simulink model "controlsystems.slx"  (R2025b)
settings: Solver=VariableStepAuto  StartTime=0.0  StopTime=50  RelTol=1e-3
libraries: simulink x1
settings Model: Creator=MANAL CHATT  LastModifiedBy=MANAL CHATT

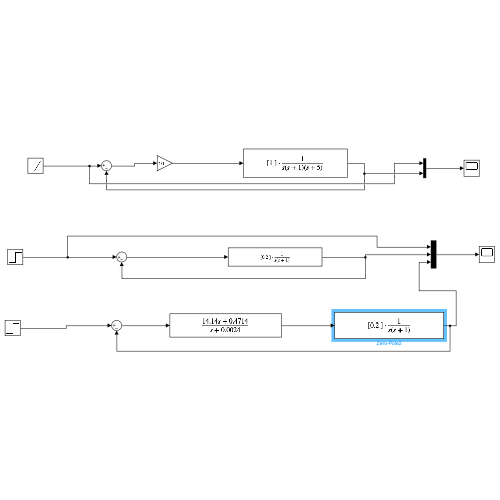
[thumbnail: Simulink's stored preview of the top-level diagram]
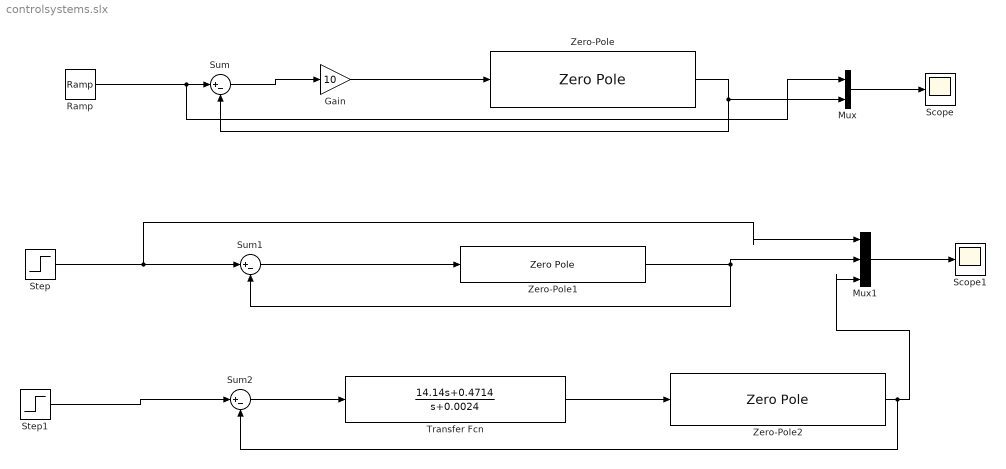
== system controlsystems.slx ==
  Gain : Gain  Gain=10
  Mux : Mux  Inputs=2
  Mux1 : Mux  Inputs=3
  Ramp : simulink/Sources/Ramp  slope=1  start=0  InitialOutput=0
  Scope : Scope
      settings: ActiveDisplayYMinimum=-6.2499999999999982  ActiveDisplayYMaximum=56.25
  Scope1 : Scope
      settings: ActiveDisplayYMinimum=-0.17289112553969113  ActiveDisplayYMaximum=1.5560201298572205
  Step : Step  SampleTime=0
  Step1 : Step  SampleTime=0
  Sum : Sum  Inputs=|+-
  Sum1 : Sum  Inputs=|+-
  Sum2 : Sum  Inputs=|+-
  Transfer Fcn : TransferFcn  Numerator=[14.14 0.4714]  Denominator=[1 0.0024]
  Zero-Pole : ZeroPole  Zeros=[]  Poles=[0 -1 -5]
  Zero-Pole1 : ZeroPole  Zeros=[]  Poles=[0 -1]  Gain=[0.2]
  Zero-Pole2 : ZeroPole  Zeros=[]  Poles=[0 -1]  Gain=[0.2]
  wires:
  Gain/1 -> Zero-Pole/1
  Zero-Pole/1 -> Mux/2, Sum/2
  Sum/1 -> Gain/1
  Mux/1 -> Scope/1
  Ramp/1 -> Mux/1, Sum/1
  Step/1 -> Mux1/1, Sum1/1
  Zero-Pole1/1 -> Sum1/2, Mux1/2
  Mux1/1 -> Scope1/1
  Sum1/1 -> Zero-Pole1/1
  Transfer Fcn/1 -> Zero-Pole2/1
  Sum2/1 -> Transfer Fcn/1
  Zero-Pole2/1 -> Sum2/2, Mux1/3
  Step1/1 -> Sum2/1
